simulink model "TENSGwithfourGFM_electromechanical"  (R2020a)
settings: Solver=VariableStepAuto  StartTime=0.0  StopTime=10.0  FixedStep=0.01  RelTol=1e-3
values from neighbouring files (symbols this model uses):
  GFMInit = GFMSimple_init(resultsac,GFM_in_gidx)    [init.m]
  GSGInit =     [SixGFMconfig.mat]    (also in eightGFMconfig.mat; fourGFMconfig.mat; init.m = SG_init(resultsac,SG_in_gidx); tenGFMconfig.mat)
  Pload = [0 0 0 0 0 0 0 0 0 0 0 0 ... (39 elements, 39x1)]    [SixGFMconfig.mat]    (also in eightGFMconfig.mat; fourGFMconfig.mat; init.m = -resultsac.bus{[CZno,CPno],3}/1000; tenGFMconfig.mat)
  Qload = -resultsac.bus{[CZno,CPno],4}/1000    [init.m]
  Satura = Ses_g(GFM_in_gidx)    [init.m]
  U = [1.0278659059 0.919047677638 0.824047236404 0.914672565668 0.984993620745 0.992890253418 1.00337242347 1.00687710353 1.06162588537 0.973548635627 0.980333735458 0.971076509646 ... (88 elements, 88x1)]    [SixGFMconfig.mat]    (also in eightGFMconfig.mat; fourGFMconfig.mat; init.m = resultsac.bus{:,8}.*exp(1i*(resultsac.bus{:,9})/180*pi); tenGFMconfig.mat)
  Vload = Vbus([CZno,CPno])    [init.m]
  W0 = wB    (= 314.159265359)    [init.m]
  Y_new = [-5.55111512313e-17 -2.77555756156e-17 0 0 0 0 0 0 0 0 0 0 ... (7744 elements, 88x88)]    [SixGFMconfig.mat]    (also in eightGFMconfig.mat; fourGFMconfig.mat; init.m = Y_new([CSno,CPno,GFMother],[CSno,CPno,GFMother]); kron.m = Y)
libraries: eeTransforms x53, simulink_extras x10
(part 2 of 3)

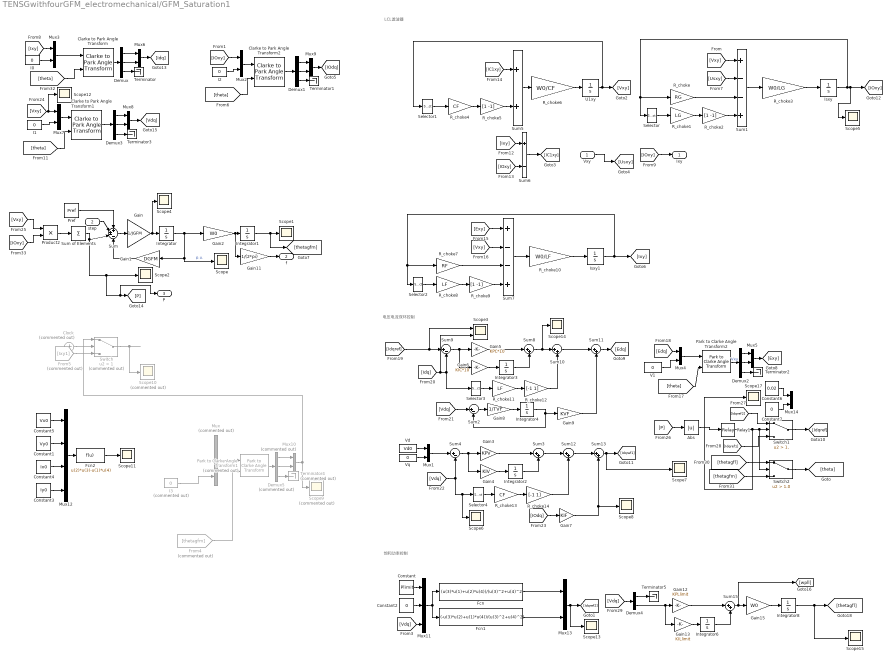
== system TENSGwithfourGFM_electromechanical/GFM_Saturation1 ==
  note: 饱和功率控制
  note: 电压电流双环控制
  note: LCL滤波器
  Vxy : Inport
  step : Inport  Port=2
  Abs : Abs
  Clarke to Park Angle Transform : eeTransforms/Clarke to Park Angle Transform  AxisAlignment=D-axis
      settings: SourceProductBaseCode=PS
  Clarke to Park Angle Transform1 : eeTransforms/Clarke to Park Angle Transform  AxisAlignment=D-axis
      settings: SourceProductBaseCode=PS
  Clarke to Park Angle Transform2 : eeTransforms/Clarke to Park Angle Transform  AxisAlignment=D-axis
      settings: SourceProductBaseCode=PS
  Clock : Clock  Commented=on
  Constant : Constant  Value=Plimit
  Constant1 : Constant  Value=Vy0
  Constant2 : Constant  Value=0
  Constant3 : Constant  Value=Iy0
  Constant4 : Constant  Value=Ix0
  Constant5 : Constant  Value=Vx0
  Constant6 : Constant  Value=0.02
  Constant7 : Constant  Value=0
  Demux{,1..3} (4 alike) : Demux  Outputs=3
  Demux4 : Demux  Outputs=2
  Demux5 : Demux  Commented=on  Outputs=3
  Fcn : Fcn  Expr=(u(3)*u(1)+u(2)*u(4))/(u(3)^2+u(4)^2)
  Fcn1 : Fcn  Expr=(-u(3)*u(2)+u(1)*u(4))/(u(3)^2+u(4)^2)
  Fcn2 : Fcn  Expr=u(2)*u(3)-u(1)*u(4)
  From4 : From  Commented=on  GotoTag=thetagfm
  From5 : From  Commented=on  GotoTag=Ixy1
  Gain : Gain  Gain=1/JGFM
  Gain1 : Gain  Gain=DGFM
  Gain11 : Gain  Gain=1/(2*pi)
  Gain12 : Gain  Gain=KPLlimit
  Gain13 : Gain  Gain=KILlimit
  Gain15 : Gain  Gain=W0
  Gain2 : Gain  Gain=W0
  Gain3 : Gain  Gain=KPV
  Gain4 : Gain  Gain=KIV
  Gain5 : Gain  Gain=KPC*10
  Gain6 : Gain  Gain=KIC*10
  Gain7 : Gain  Gain=KIF
  Gain8 : Gain  Gain=1/TVF
  Gain9 : Gain  Gain=KVF
  I0 : Constant  Value=0
  I1 : Constant  Value=0
  I2 : Constant  Value=0
  I3 : Constant  Commented=on  Value=0
  Integrator : Integrator
  Integrator1 : Integrator  InitialCondition=theta0
  Integrator2 : Integrator  InitialCondition=[Idref0 Iqref0]
  Integrator3 : Integrator  InitialCondition=[Ed0 Eq0]
  Integrator4 : Integrator  InitialCondition=[Vd0 0]
  Integrator6 : Integrator
  Integrator8 : Integrator  InitialCondition=theta0
  Isxy : Integrator  InitialCondition=[IOx0 IOy0]
  Isxy1 : Integrator  InitialCondition=[Ix0 Iy0]
  Mux : Mux  Commented=on  Inputs=3
  Mux{1..9,13..14} (11 alike) : Mux  Inputs=2
  Mux10 : Mux  Commented=on  Inputs=2
  Mux11 : Mux  Inputs=3
  Mux12 : Mux
  Park to Clarke Angle Transform1 : eeTransforms/Park to Clarke Angle Transform  Commented=on  AxisAlignment=D-axis
      settings: SourceProductBaseCode=PS
  Park to Clarke Angle Transform2 : eeTransforms/Park to Clarke Angle Transform  AxisAlignment=D-axis
      settings: SourceProductBaseCode=PS
  Pref : Constant  Value=Pref
  Product2 : Product
  R_choke : Gain  Gain=RG  SaturateOnIntegerOverflow=on  OutDataTypeStr=Inherit: Same as input  ParamDataTypeStr=Inherit: Same as input
  R_choke1 : Gain  Gain=LG  SaturateOnIntegerOverflow=on  OutDataTypeStr=Inherit: Same as input  ParamDataTypeStr=Inherit: Same as input
  R_choke10 : Gain  Gain=W0/LF  SaturateOnIntegerOverflow=on  OutDataTypeStr=Inherit: Same as input  ParamDataTypeStr=Inherit: Same as input
  R_choke11 : Gain  Gain=LF  SaturateOnIntegerOverflow=on  OutDataTypeStr=Inherit: Same as input  ParamDataTypeStr=Inherit: Same as input
  R_choke12 : Gain  Gain=[-1 1]  SaturateOnIntegerOverflow=on  OutDataTypeStr=Inherit: Same as input  ParamDataTypeStr=Inherit: Same as input
  R_choke13 : Gain  Gain=CF  SaturateOnIntegerOverflow=on  OutDataTypeStr=Inherit: Same as input  ParamDataTypeStr=Inherit: Same as input
  R_choke14 : Gain  Gain=[-1 1]  SaturateOnIntegerOverflow=on  OutDataTypeStr=Inherit: Same as input  ParamDataTypeStr=Inherit: Same as input
  R_choke2 : Gain  Gain=[1 -1]  SaturateOnIntegerOverflow=on  OutDataTypeStr=Inherit: Same as input  ParamDataTypeStr=Inherit: Same as input
  R_choke3 : Gain  Gain=W0/LG  SaturateOnIntegerOverflow=on  OutDataTypeStr=Inherit: Same as input  ParamDataTypeStr=Inherit: Same as input
  R_choke4 : Gain  Gain=CF  SaturateOnIntegerOverflow=on  OutDataTypeStr=Inherit: Same as input  ParamDataTypeStr=Inherit: Same as input
  R_choke5 : Gain  Gain=[1 -1]  SaturateOnIntegerOverflow=on  OutDataTypeStr=Inherit: Same as input  ParamDataTypeStr=Inherit: Same as input
  R_choke6 : Gain  Gain=W0/CF  SaturateOnIntegerOverflow=on  OutDataTypeStr=Inherit: Same as input  ParamDataTypeStr=Inherit: Same as input
  R_choke7 : Gain  Gain=RF  SaturateOnIntegerOverflow=on  OutDataTypeStr=Inherit: Same as input  ParamDataTypeStr=Inherit: Same as input
  R_choke8 : Gain  Gain=LF  SaturateOnIntegerOverflow=on  OutDataTypeStr=Inherit: Same as input  ParamDataTypeStr=Inherit: Same as input
  R_choke9 : Gain  Gain=[1 -1]  SaturateOnIntegerOverflow=on  OutDataTypeStr=Inherit: Same as input  ParamDataTypeStr=Inherit: Same as input
  Relay1 : Relay  OnSwitchValue=Plimit  OffSwitchValue=0  OnOutputValue=1.1
  Scope{,1..2,4..8,11..15,17} (14 alike) : Scope
  Scope10 : Scope  Commented=on
  Scope3 : Scope  NumInputPorts=2
  Scope9 : Scope  Commented=on
  Selector{,1..4} (5 alike) : Selector  InputPortWidth=2  IndexOptions=Index vector (dialog)  Indices=[2 1]  OutputSizes=1
  Sum : Sum  Inputs=++--
  Sum of Elements : Sum  Inputs=+
  Sum1 : Sum  Inputs=+--+  SaturateOnIntegerOverflow=on
  Sum{3,8,10..13,15} (7 alike) : Sum  Inputs=|++
  Sum2 : Sum  Inputs=|+-
  Sum4 : Sum  Inputs=|+-
  Sum5 : Sum  SaturateOnIntegerOverflow=on
  Sum6 : Sum  Inputs=+-  SaturateOnIntegerOverflow=on
  Sum7 : Sum  Inputs=+--+  SaturateOnIntegerOverflow=on
  Sum9 : Sum  Inputs=|+-
  Switch : Switch  Commented=on  Criteria=u2 > Threshold  Threshold=1
  Switch1 : Switch  Criteria=u2 > Threshold  Threshold=1.
  Switch2 : Switch  Criteria=u2 > Threshold  Threshold=1.0
  Terminator{,1..3,5} (5 alike) : Terminator
  Terminator4 : Terminator  Commented=on
  U1xy : Integrator  InitialCondition=[Vx0 Vy0]
  V1 : Constant  Value=0
  Vd : Constant  Value=Vd0
  Vq : Constant  Value=0
  Ixy : Outport
  f : Outport  Port=2
  P : Outport  Port=3
  wires:
  Integrator1/1 -> [thetagfm], Scope1/1
  Mux3/1 -> Clarke to Park Angle Transform/1
  I0/1 -> Mux3/2
  Demux/3 -> Terminator/1
  Demux/2 -> Mux6/2
  Gain/1 -> Scope4/1, Integrator/1
  Demux/1 -> Mux6/1
  Clarke to Park Angle Transform/1 -> Demux/1
  Integrator/1 -> Gain2/1, Scope/1, Gain1/1  "p.u."
  Sum of Elements/1 -> Sum/3, P/1, [P], Scope2/1
  Sum/1 -> Gain/1
  Vxy/1 -> [Usxy]
  [Vxy] -> Sum1/1
  [Usxy] -> Sum1/2
  Sum1/1 -> R_choke3/1
  R_choke3/1 -> Isxy/1
  R_choke1/1 -> R_choke2/1
  Isxy/1 -> Scope5/1, [IOxy], R_choke/1, Selector/1
  R_choke/1 -> Sum1/3
  Selector/1 -> R_choke1/1
  R_choke2/1 -> Sum1/4
  [Ixy] -> Mux3/1
  [IOxy] -> Ixy/1
  [theta] -> Clarke to Park Angle Transform/2
  Gain4/1 -> Integrator2/1
  Sum3/1 -> Sum12/1
  Gain3/1 -> Sum3/1
  Integrator2/1 -> Sum3/2
  Sum4/1 -> Gain4/1, Gain3/1
  Vd/1 -> Mux1/1
  Vq/1 -> Mux1/2
  Mux1/1 -> Sum4/1
  R_choke4/1 -> R_choke5/1
  R_choke5/1 -> Sum5/2
  Sum6/1 -> [IC1xy]
  U1xy/1 -> Selector1/1, [Vxy]
  R_choke6/1 -> U1xy/1
  [Ixy] -> Sum6/1
  Selector1/1 -> R_choke4/1
  [IOxy] -> Sum6/2
  [IC1xy] -> Sum5/1
  Sum5/1 -> R_choke6/1
  Isxy1/1 -> [Ixy], R_choke7/1, Selector2/1
  [Vxy] -> Sum7/2
  R_choke7/1 -> Sum7/3
  R_choke8/1 -> R_choke9/1
  R_choke10/1 -> Isxy1/1
  Sum7/1 -> R_choke10/1
  R_choke9/1 -> Sum7/4
  Selector2/1 -> R_choke8/1
  [Edq] -> Mux4/1
  V1/1 -> Mux4/2
  Mux4/1 -> Park to Clarke Angle Transform2/1
  [theta] -> Park to Clarke Angle Transform2/2
  Mux5/1 -> [Exy]
  Demux2/3 -> Terminator2/1
  Park to Clarke Angle Transform2/1 -> Demux2/1  "Vxy"
  Demux2/2 -> Mux5/2
  Demux2/1 -> Mux5/1
  Sum9/1 -> Gain6/1, Gain5/1
  Gain5/1 -> Sum8/1
  Gain6/1 -> Integrator3/1
  Integrator3/1 -> Sum8/2
  R_choke11/1 -> R_choke12/1
  Selector3/1 -> R_choke11/1
  Sum8/1 -> Scope14/1, Sum10/1
  R_choke12/1 -> Sum10/2
  Sum10/1 -> Sum11/1
  Gain9/1 -> Sum11/2
  Sum11/1 -> [Edq]
  Selector4/1 -> R_choke13/1
  [Vdq] -> Scope6/1, Selector4/1, Sum4/2
  R_choke13/1 -> R_choke14/1
  R_choke14/1 -> Sum12/2
  Sum12/1 -> Sum13/1
  Sum13/1 -> Scope7/1, [Idqref1]
  [IOdq] -> Gain7/1
  Gain7/1 -> Sum13/2, Scope8/1
  Mux6/1 -> [Idq]
  [Vxy] -> Scope12/1, Mux7/1
  I1/1 -> Mux7/2
  Mux7/1 -> Clarke to Park Angle Transform1/1
  [theta] -> Clarke to Park Angle Transform1/2
  Clarke to Park Angle Transform1/1 -> Demux3/1
  Demux3/1 -> Mux8/1
  Demux3/2 -> Mux8/2
  Mux8/1 -> [Vdq]
  Demux3/3 -> Terminator3/1
  [theta] -> Clarke to Park Angle Transform2/2
  Clarke to Park Angle Transform2/1 -> Demux1/1
  Demux1/1 -> Mux9/1
  Demux1/2 -> Mux9/2
  [IOxy] -> Mux2/1
  Demux1/3 -> Terminator1/1
  Mux2/1 -> Clarke to Park Angle Transform2/1
  Mux9/1 -> [IOdq]
  I2/1 -> Mux2/2
  [Vxy] -> Product2/1
  [IOxy] -> Product2/2
  Product2/1 -> Sum of Elements/1
  Sum2/1 -> Gain8/1
  Integrator4/1 -> Gain9/1, Sum2/2
  Gain8/1 -> Integrator4/1
  [Vdq] -> Sum2/1
  [Exy] -> Sum7/1
  Gain2/1 -> Gain11/1, Integrator1/1
  Gain11/1 -> f/1
  Pref/1 -> Sum/1
  [Idq] -> Sum9/2, Selector3/1, Scope3/2
  Demux5/3 -> Terminator4/1
  Mux/1 -> Park to Clarke Angle Transform1/1
  Demux5/2 -> Mux10/2
  Park to Clarke Angle Transform1/1 -> Demux5/1
  Mux10/1 -> Scope9/1, Switch/1
  Demux5/1 -> Mux10/1
  I3/1 -> Mux/3
  [Idqref] -> Scope3/1, Sum9/1
  Switch/1 -> Scope10/1
  From5/1 -> Switch/3
  Clock/1 -> Switch/2
  From4/1 -> Park to Clarke Angle Transform1/2
  Mux11/1 -> Fcn1/1, Fcn/1
  Constant/1 -> Mux11/1
  Constant5/1 -> Mux12/1
  Constant1/1 -> Mux12/2
  Constant4/1 -> Mux12/3
  Constant3/1 -> Mux12/4
  Mux12/1 -> Fcn2/1
  Constant2/1 -> Mux11/2
  Fcn2/1 -> Scope11/1
  Mux13/1 -> Scope13/1, [Idqref2]
  [P] -> Abs/1
  Relay1/1 -> Scope17/1, Switch1/2, Switch2/2
  Switch1/1 -> [Idqref]
  [Idqref1] -> Switch1/3
  Integrator6/1 -> Sum15/2
  Gain13/1 -> Integrator6/1
  Demux4/1 -> Terminator5/1
  Gain15/1 -> Integrator8/1
  [Vdq] -> Demux4/1
  Demux4/2 -> Gain13/1, Gain12/1
  Integrator8/1 -> Scope15/1, [thetagfl]
  Gain12/1 -> Sum15/1
  [thetagfl] -> Switch2/1
  [thetagfm] -> Switch2/3
  Switch2/1 -> [theta]
  Fcn/1 -> Mux13/1
  Fcn1/1 -> Mux13/2
  [Vdq] -> Mux11/3
  Constant6/1 -> Mux14/1
  Constant7/1 -> Mux14/2
  [Idqref2] -> Switch1/1
  Sum15/1 -> [wpll], Gain15/1
  Abs/1 -> Relay1/1
  Gain1/1 -> Sum/4
  step/1 -> Sum/2

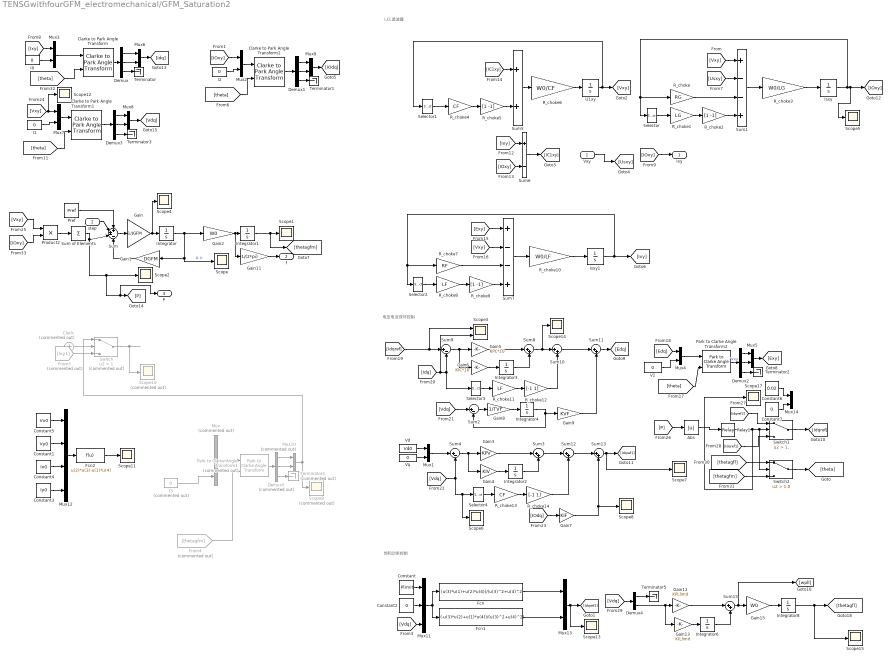
== system TENSGwithfourGFM_electromechanical/GFM_Saturation2 ==
  note: LCL滤波器
  note: 电压电流双环控制
  note: 饱和功率控制
  Vxy : Inport
  step : Inport  Port=2
  Abs : Abs
  Clarke to Park Angle Transform : eeTransforms/Clarke to Park Angle Transform  AxisAlignment=D-axis
      settings: SourceProductBaseCode=PS
  Clarke to Park Angle Transform1 : eeTransforms/Clarke to Park Angle Transform  AxisAlignment=D-axis
      settings: SourceProductBaseCode=PS
  Clarke to Park Angle Transform2 : eeTransforms/Clarke to Park Angle Transform  AxisAlignment=D-axis
      settings: SourceProductBaseCode=PS
  Clock : Clock  Commented=on
  Constant : Constant  Value=Plimit
  Constant1 : Constant  Value=Vy0
  Constant2 : Constant  Value=0
  Constant3 : Constant  Value=Iy0
  Constant4 : Constant  Value=Ix0
  Constant5 : Constant  Value=Vx0
  Constant6 : Constant  Value=0.02
  Constant7 : Constant  Value=0
  Demux{,1..3} (4 alike) : Demux  Outputs=3
  Demux4 : Demux  Outputs=2
  Demux5 : Demux  Commented=on  Outputs=3
  Fcn : Fcn  Expr=(u(3)*u(1)+u(2)*u(4))/(u(3)^2+u(4)^2)
  Fcn1 : Fcn  Expr=(-u(3)*u(2)+u(1)*u(4))/(u(3)^2+u(4)^2)
  Fcn2 : Fcn  Expr=u(2)*u(3)-u(1)*u(4)
  From4 : From  Commented=on  GotoTag=thetagfm
  From5 : From  Commented=on  GotoTag=Ixy1
  Gain : Gain  Gain=1/JGFM
  Gain1 : Gain  Gain=DGFM
  Gain11 : Gain  Gain=1/(2*pi)
  Gain12 : Gain  Gain=KPLlimit
  Gain13 : Gain  Gain=KILlimit
  Gain15 : Gain  Gain=W0
  Gain2 : Gain  Gain=W0
  Gain3 : Gain  Gain=KPV
  Gain4 : Gain  Gain=KIV
  Gain5 : Gain  Gain=KPC*10
  Gain6 : Gain  Gain=KIC*10
  Gain7 : Gain  Gain=KIF
  Gain8 : Gain  Gain=1/TVF
  Gain9 : Gain  Gain=KVF
  I0 : Constant  Value=0
  I1 : Constant  Value=0
  I2 : Constant  Value=0
  I3 : Constant  Commented=on  Value=0
  Integrator : Integrator
  Integrator1 : Integrator  InitialCondition=theta0
  Integrator2 : Integrator  InitialCondition=[Idref0 Iqref0]
  Integrator3 : Integrator  InitialCondition=[Ed0 Eq0]
  Integrator4 : Integrator  InitialCondition=[Vd0 0]
  Integrator6 : Integrator
  Integrator8 : Integrator  InitialCondition=theta0
  Isxy : Integrator  InitialCondition=[IOx0 IOy0]
  Isxy1 : Integrator  InitialCondition=[Ix0 Iy0]
  Mux : Mux  Commented=on  Inputs=3
  Mux{1..9,13..14} (11 alike) : Mux  Inputs=2
  Mux10 : Mux  Commented=on  Inputs=2
  Mux11 : Mux  Inputs=3
  Mux12 : Mux
  Park to Clarke Angle Transform1 : eeTransforms/Park to Clarke Angle Transform  Commented=on  AxisAlignment=D-axis
      settings: SourceProductBaseCode=PS
  Park to Clarke Angle Transform2 : eeTransforms/Park to Clarke Angle Transform  AxisAlignment=D-axis
      settings: SourceProductBaseCode=PS
  Pref : Constant  Value=Pref
  Product2 : Product
  R_choke : Gain  Gain=RG  SaturateOnIntegerOverflow=on  OutDataTypeStr=Inherit: Same as input  ParamDataTypeStr=Inherit: Same as input
  R_choke1 : Gain  Gain=LG  SaturateOnIntegerOverflow=on  OutDataTypeStr=Inherit: Same as input  ParamDataTypeStr=Inherit: Same as input
  R_choke10 : Gain  Gain=W0/LF  SaturateOnIntegerOverflow=on  OutDataTypeStr=Inherit: Same as input  ParamDataTypeStr=Inherit: Same as input
  R_choke11 : Gain  Gain=LF  SaturateOnIntegerOverflow=on  OutDataTypeStr=Inherit: Same as input  ParamDataTypeStr=Inherit: Same as input
  R_choke12 : Gain  Gain=[-1 1]  SaturateOnIntegerOverflow=on  OutDataTypeStr=Inherit: Same as input  ParamDataTypeStr=Inherit: Same as input
  R_choke13 : Gain  Gain=CF  SaturateOnIntegerOverflow=on  OutDataTypeStr=Inherit: Same as input  ParamDataTypeStr=Inherit: Same as input
  R_choke14 : Gain  Gain=[-1 1]  SaturateOnIntegerOverflow=on  OutDataTypeStr=Inherit: Same as input  ParamDataTypeStr=Inherit: Same as input
  R_choke2 : Gain  Gain=[1 -1]  SaturateOnIntegerOverflow=on  OutDataTypeStr=Inherit: Same as input  ParamDataTypeStr=Inherit: Same as input
  R_choke3 : Gain  Gain=W0/LG  SaturateOnIntegerOverflow=on  OutDataTypeStr=Inherit: Same as input  ParamDataTypeStr=Inherit: Same as input
  R_choke4 : Gain  Gain=CF  SaturateOnIntegerOverflow=on  OutDataTypeStr=Inherit: Same as input  ParamDataTypeStr=Inherit: Same as input
  R_choke5 : Gain  Gain=[1 -1]  SaturateOnIntegerOverflow=on  OutDataTypeStr=Inherit: Same as input  ParamDataTypeStr=Inherit: Same as input
  R_choke6 : Gain  Gain=W0/CF  SaturateOnIntegerOverflow=on  OutDataTypeStr=Inherit: Same as input  ParamDataTypeStr=Inherit: Same as input
  R_choke7 : Gain  Gain=RF  SaturateOnIntegerOverflow=on  OutDataTypeStr=Inherit: Same as input  ParamDataTypeStr=Inherit: Same as input
  R_choke8 : Gain  Gain=LF  SaturateOnIntegerOverflow=on  OutDataTypeStr=Inherit: Same as input  ParamDataTypeStr=Inherit: Same as input
  R_choke9 : Gain  Gain=[1 -1]  SaturateOnIntegerOverflow=on  OutDataTypeStr=Inherit: Same as input  ParamDataTypeStr=Inherit: Same as input
  Relay1 : Relay  OnSwitchValue=Plimit  OffSwitchValue=0  OnOutputValue=1.1
  Scope{,1..2,4..8,11..15,17} (14 alike) : Scope
  Scope10 : Scope  Commented=on
  Scope3 : Scope  NumInputPorts=2
  Scope9 : Scope  Commented=on
  Selector{,1..4} (5 alike) : Selector  InputPortWidth=2  IndexOptions=Index vector (dialog)  Indices=[2 1]  OutputSizes=1
  Sum : Sum  Inputs=++--
  Sum of Elements : Sum  Inputs=+
  Sum1 : Sum  Inputs=+--+  SaturateOnIntegerOverflow=on
  Sum{3,8,10..13,15} (7 alike) : Sum  Inputs=|++
  Sum2 : Sum  Inputs=|+-
  Sum4 : Sum  Inputs=|+-
  Sum5 : Sum  SaturateOnIntegerOverflow=on
  Sum6 : Sum  Inputs=+-  SaturateOnIntegerOverflow=on
  Sum7 : Sum  Inputs=+--+  SaturateOnIntegerOverflow=on
  Sum9 : Sum  Inputs=|+-
  Switch : Switch  Commented=on  Criteria=u2 > Threshold  Threshold=1
  Switch1 : Switch  Criteria=u2 > Threshold  Threshold=1.
  Switch2 : Switch  Criteria=u2 > Threshold  Threshold=1.0
  Terminator{,1..3,5} (5 alike) : Terminator
  Terminator4 : Terminator  Commented=on
  U1xy : Integrator  InitialCondition=[Vx0 Vy0]
  V1 : Constant  Value=0
  Vd : Constant  Value=Vd0
  Vq : Constant  Value=0
  Ixy : Outport
  f : Outport  Port=2
  P : Outport  Port=3
  wires:
  step/1 -> Sum/2
  Gain1/1 -> Sum/4
  Abs/1 -> Relay1/1
  Sum15/1 -> Gain15/1, [wpll]
  [Idqref2] -> Switch1/1
  Constant7/1 -> Mux14/2
  Constant6/1 -> Mux14/1
  [Vdq] -> Mux11/3
  Fcn1/1 -> Mux13/2
  Fcn/1 -> Mux13/1
  Switch2/1 -> [theta]
  [thetagfm] -> Switch2/3
  [thetagfl] -> Switch2/1
  Gain12/1 -> Sum15/1
  Integrator8/1 -> [thetagfl], Scope15/1
  Demux4/2 -> Gain12/1, Gain13/1
  [Vdq] -> Demux4/1
  Gain15/1 -> Integrator8/1
  Demux4/1 -> Terminator5/1
  Gain13/1 -> Integrator6/1
  Integrator6/1 -> Sum15/2
  [Idqref1] -> Switch1/3
  Switch1/1 -> [Idqref]
  Relay1/1 -> Switch2/2, Switch1/2, Scope17/1
  [P] -> Abs/1
  Mux13/1 -> [Idqref2], Scope13/1
  Fcn2/1 -> Scope11/1
  Constant2/1 -> Mux11/2
  Mux12/1 -> Fcn2/1
  Constant3/1 -> Mux12/4
  Constant4/1 -> Mux12/3
  Constant1/1 -> Mux12/2
  Constant5/1 -> Mux12/1
  Constant/1 -> Mux11/1
  Mux11/1 -> Fcn/1, Fcn1/1
  From4/1 -> Park to Clarke Angle Transform1/2
  Clock/1 -> Switch/2
  From5/1 -> Switch/3
  Switch/1 -> Scope10/1
  [Idqref] -> Sum9/1, Scope3/1
  I3/1 -> Mux/3
  Demux5/1 -> Mux10/1
  Mux10/1 -> Switch/1, Scope9/1
  Park to Clarke Angle Transform1/1 -> Demux5/1
  Demux5/2 -> Mux10/2
  Mux/1 -> Park to Clarke Angle Transform1/1
  Demux5/3 -> Terminator4/1
  [Idq] -> Scope3/2, Selector3/1, Sum9/2
  Pref/1 -> Sum/1
  Gain11/1 -> f/1
  Gain2/1 -> Integrator1/1, Gain11/1
  [Exy] -> Sum7/1
  [Vdq] -> Sum2/1
  Gain8/1 -> Integrator4/1
  Integrator4/1 -> Sum2/2, Gain9/1
  Sum2/1 -> Gain8/1
  Product2/1 -> Sum of Elements/1
  [IOxy] -> Product2/2
  [Vxy] -> Product2/1
  I2/1 -> Mux2/2
  Mux9/1 -> [IOdq]
  Mux2/1 -> Clarke to Park Angle Transform2/1
  Demux1/3 -> Terminator1/1
  [IOxy] -> Mux2/1
  Demux1/2 -> Mux9/2
  Demux1/1 -> Mux9/1
  Clarke to Park Angle Transform2/1 -> Demux1/1
  [theta] -> Clarke to Park Angle Transform2/2
  Demux3/3 -> Terminator3/1
  Mux8/1 -> [Vdq]
  Demux3/2 -> Mux8/2
  Demux3/1 -> Mux8/1
  Clarke to Park Angle Transform1/1 -> Demux3/1
  [theta] -> Clarke to Park Angle Transform1/2
  Mux7/1 -> Clarke to Park Angle Transform1/1
  I1/1 -> Mux7/2
  [Vxy] -> Mux7/1, Scope12/1
  Mux6/1 -> [Idq]
  Gain7/1 -> Scope8/1, Sum13/2
  [IOdq] -> Gain7/1
  Sum13/1 -> [Idqref1], Scope7/1
  Sum12/1 -> Sum13/1
  R_choke14/1 -> Sum12/2
  R_choke13/1 -> R_choke14/1
  [Vdq] -> Sum4/2, Selector4/1, Scope6/1
  Selector4/1 -> R_choke13/1
  Sum11/1 -> [Edq]
  Gain9/1 -> Sum11/2
  Sum10/1 -> Sum11/1
  R_choke12/1 -> Sum10/2
  Sum8/1 -> Sum10/1, Scope14/1
  Selector3/1 -> R_choke11/1
  R_choke11/1 -> R_choke12/1
  Integrator3/1 -> Sum8/2
  Gain6/1 -> Integrator3/1
  Gain5/1 -> Sum8/1
  Sum9/1 -> Gain5/1, Gain6/1
  Demux2/1 -> Mux5/1
  Demux2/2 -> Mux5/2
  Park to Clarke Angle Transform2/1 -> Demux2/1  "Vxy"
  Demux2/3 -> Terminator2/1
  Mux5/1 -> [Exy]
  [theta] -> Park to Clarke Angle Transform2/2
  Mux4/1 -> Park to Clarke Angle Transform2/1
  V1/1 -> Mux4/2
  [Edq] -> Mux4/1
  Selector2/1 -> R_choke8/1
  R_choke9/1 -> Sum7/4
  Sum7/1 -> R_choke10/1
  R_choke10/1 -> Isxy1/1
  R_choke8/1 -> R_choke9/1
  R_choke7/1 -> Sum7/3
  [Vxy] -> Sum7/2
  Isxy1/1 -> Selector2/1, R_choke7/1, [Ixy]
  Sum5/1 -> R_choke6/1
  [IC1xy] -> Sum5/1
  [IOxy] -> Sum6/2
  Selector1/1 -> R_choke4/1
  [Ixy] -> Sum6/1
  R_choke6/1 -> U1xy/1
  U1xy/1 -> [Vxy], Selector1/1
  Sum6/1 -> [IC1xy]
  R_choke5/1 -> Sum5/2
  R_choke4/1 -> R_choke5/1
  Mux1/1 -> Sum4/1
  Vq/1 -> Mux1/2
  Vd/1 -> Mux1/1
  Sum4/1 -> Gain3/1, Gain4/1
  Integrator2/1 -> Sum3/2
  Gain3/1 -> Sum3/1
  Sum3/1 -> Sum12/1
  Gain4/1 -> Integrator2/1
  [theta] -> Clarke to Park Angle Transform/2
  [IOxy] -> Ixy/1
  [Ixy] -> Mux3/1
  R_choke2/1 -> Sum1/4
  Selector/1 -> R_choke1/1
  R_choke/1 -> Sum1/3
  Isxy/1 -> Selector/1, R_choke/1, [IOxy], Scope5/1
  R_choke1/1 -> R_choke2/1
  R_choke3/1 -> Isxy/1
  Sum1/1 -> R_choke3/1
  [Usxy] -> Sum1/2
  [Vxy] -> Sum1/1
  Vxy/1 -> [Usxy]
  Sum/1 -> Gain/1
  Sum of Elements/1 -> Scope2/1, [P], P/1, Sum/3
  Integrator/1 -> Gain1/1, Scope/1, Gain2/1  "p.u."
  Clarke to Park Angle Transform/1 -> Demux/1
  Demux/1 -> Mux6/1
  Gain/1 -> Integrator/1, Scope4/1
  Demux/2 -> Mux6/2
  Demux/3 -> Terminator/1
  I0/1 -> Mux3/2
  Mux3/1 -> Clarke to Park Angle Transform/1
  Integrator1/1 -> Scope1/1, [thetagfm]

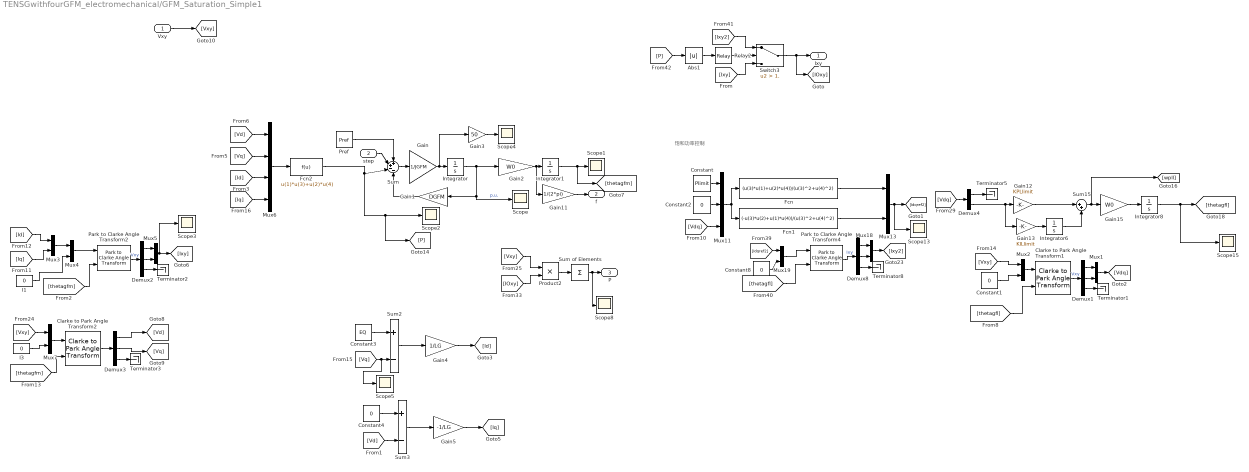
== system TENSGwithfourGFM_electromechanical/GFM_Saturation_Simple1 ==
  note: 饱和功率控制
  Vxy : Inport
  step : Inport  Port=2
  Abs1 : Abs
  Clarke to Park Angle Transform1 : eeTransforms/Clarke to Park Angle Transform  AxisAlignment=D-axis
      settings: SourceProductBaseCode=PS
  Clarke to Park Angle Transform2 : eeTransforms/Clarke to Park Angle Transform  AxisAlignment=D-axis
      settings: SourceProductBaseCode=PS
  Constant : Constant  Value=Plimit
  Constant{1..2,4,8} (4 alike) : Constant  Value=0
  Constant3 : Constant  Value=EQ
  Demux{1..3,8} (4 alike) : Demux  Outputs=3
  Demux4 : Demux  Outputs=2
  Fcn : Fcn  Expr=(u(3)*u(1)+u(2)*u(4))/(u(3)^2+u(4)^2)
  Fcn1 : Fcn  Expr=(-u(3)*u(2)+u(1)*u(4))/(u(3)^2+u(4)^2)
  Fcn2 : Fcn  Expr=u(1)*u(3)+u(2)*u(4)
  Gain : Gain  Gain=1/JGFM
  Gain1 : Gain  Gain=DGFM
  Gain11 : Gain  Gain=1/(2*pi)
  Gain12 : Gain  Gain=KPLlimit
  Gain13 : Gain  Gain=KILlimit
  Gain15 : Gain  Gain=W0
  Gain2 : Gain  Gain=W0
  Gain3 : Gain  Gain=50
  Gain4 : Gain  Gain=1/LG
  Gain5 : Gain  Gain=-1/LG
  I1 : Constant  Value=0
  I3 : Constant  Value=0
  Integrator : Integrator
  Integrator1 : Integrator  InitialCondition=theta0
  Integrator6 : Integrator
  Integrator8 : Integrator  InitialCondition=theta0
  Mux{1..5,7,13,18..19} (9 alike) : Mux  Inputs=2
  Mux11 : Mux  Inputs=3
  Mux6 : Mux
  Park to Clarke Angle Transform2 : eeTransforms/Park to Clarke Angle Transform  AxisAlignment=D-axis
      settings: SourceProductBaseCode=PS
  Park to Clarke Angle Transform4 : eeTransforms/Park to Clarke Angle Transform  AxisAlignment=D-axis
      settings: SourceProductBaseCode=PS
  Pref : Constant  Value=Pref
  Product2 : Product
  Relay2 : Relay  OnSwitchValue=Plimit  OffSwitchValue=0  OnOutputValue=1.1
  Scope{,1..5,8,13,15} (9 alike) : Scope
  Sum : Sum  Inputs=++--
  Sum of Elements : Sum  Inputs=+
  Sum15 : Sum  Inputs=|++
  Sum2 : Sum  Inputs=+-  SaturateOnIntegerOverflow=on
  Sum3 : Sum  Inputs=+-  SaturateOnIntegerOverflow=on
  Switch3 : Switch  Criteria=u2 > Threshold  Threshold=1.
  Terminator{1..3,5,8} (5 alike) : Terminator
  Ixy : Outport
  f : Outport  Port=2
  P : Outport  Port=3
  wires:
  Integrator1/1 -> [thetagfm], Scope1/1
  Gain/1 -> Gain3/1, Integrator/1
  Integrator/1 -> Gain2/1, Scope/1, Gain1/1  "p.u."
  Fcn2/1 -> Sum/3, [P], Scope2/1
  Sum/1 -> Gain/1
  Vxy/1 -> [Vxy]
  Gain2/1 -> Gain11/1, Integrator1/1
  Gain11/1 -> f/1
  Pref/1 -> Sum/1
  Mux11/1 -> Fcn1/1, Fcn/1
  Constant/1 -> Mux11/1
  Constant2/1 -> Mux11/2
  Mux13/1 -> Scope13/1, [Idqref2]
  Integrator6/1 -> Sum15/2
  Gain13/1 -> Integrator6/1
  Demux4/1 -> Terminator5/1
  Gain15/1 -> Integrator8/1
  [Vdq] -> Demux4/1
  Demux4/2 -> Gain13/1, Gain12/1
  Integrator8/1 -> Scope15/1, [thetagfl]
  Gain12/1 -> Sum15/1
  Fcn/1 -> Mux13/1
  Fcn1/1 -> Mux13/2
  [Vdq] -> Mux11/3
  Sum15/1 -> [wpll], Gain15/1
  Gain1/1 -> Sum/4
  step/1 -> Sum/2
  Demux8/3 -> Terminator8/1
  Mux18/1 -> [Ixy2]
  Park to Clarke Angle Transform4/1 -> Demux8/1  "Ixy"
  Demux8/2 -> Mux18/2
  Demux8/1 -> Mux18/1
  [Idqref2] -> Mux19/1
  Constant8/1 -> Mux19/2
  Mux19/1 -> Park to Clarke Angle Transform4/1
  [thetagfl] -> Park to Clarke Angle Transform4/2
  [P] -> Abs1/1
  Abs1/1 -> Relay2/1
  Relay2/1 -> Switch3/2
  [Ixy2] -> Switch3/1
  [Ixy] -> Switch3/3
  Switch3/1 -> [IOxy], Ixy/1
  [Vxy] -> Mux2/1
  Constant1/1 -> Mux2/2
  Mux2/1 -> Clarke to Park Angle Transform1/1
  [thetagfl] -> Clarke to Park Angle Transform1/2
  Demux1/3 -> Terminator1/1
  Mux1/1 -> [Vdq]
  Clarke to Park Angle Transform1/1 -> Demux1/1  "Vxy"
  Demux1/2 -> Mux1/2
  Demux1/1 -> Mux1/1
  Gain3/1 -> Scope4/1
  Constant3/1 -> Sum2/1
  [Vq] -> Scope5/1, Sum2/2
  Sum2/1 -> Gain4/1
  Gain4/1 -> [Id]
  Sum3/1 -> Gain5/1
  Constant4/1 -> Sum3/1
  [Vd] -> Sum3/2
  Gain5/1 -> [Iq]
  Demux2/3 -> Terminator2/1
  Demux3/1 -> [Vd]
  [thetagfm] -> Clarke to Park Angle Transform2/2
  Park to Clarke Angle Transform2/1 -> Demux2/1  "Vxy"
  Demux2/2 -> Mux5/2
  Mux4/1 -> Park to Clarke Angle Transform2/1
  Demux3/2 -> [Vq]
  Demux3/3 -> Terminator3/1
  I3/1 -> Mux7/2
  Demux2/1 -> Mux5/1
  Clarke to Park Angle Transform2/1 -> Demux3/1
  Mux5/1 -> [Ixy], Scope3/1
  [thetagfm] -> Park to Clarke Angle Transform2/2
  [Vxy] -> Mux7/1
  Mux7/1 -> Clarke to Park Angle Transform2/1
  [Id] -> Mux3/1
  [Iq] -> Mux3/2
  Mux3/1 -> Mux4/1
  I1/1 -> Mux4/2
  [Id] -> Mux6/3
  [Vd] -> Mux6/1
  Mux6/1 -> Fcn2/1
  [Vq] -> Mux6/2
  [Iq] -> Mux6/4
  [IOxy] -> Product2/2
  Product2/1 -> Sum of Elements/1
  Sum of Elements/1 -> Scope8/1, P/1
  [Vxy] -> Product2/1

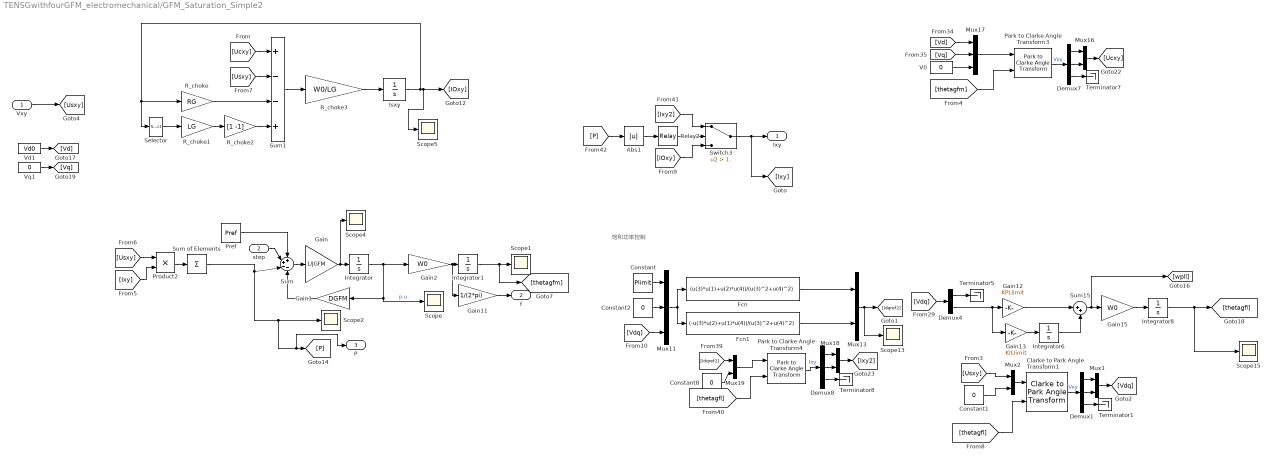
== system TENSGwithfourGFM_electromechanical/GFM_Saturation_Simple2 ==
  note: 饱和功率控制
  Vxy : Inport
  step : Inport  Port=2
  Abs1 : Abs
  Clarke to Park Angle Transform1 : eeTransforms/Clarke to Park Angle Transform  AxisAlignment=D-axis
      settings: SourceProductBaseCode=PS
  Constant : Constant  Value=Plimit
  Constant1 : Constant  Value=0
  Constant2 : Constant  Value=0
  Constant8 : Constant  Value=0
  Demux1 : Demux  Outputs=3
  Demux4 : Demux  Outputs=2
  Demux7 : Demux  Outputs=3
  Demux8 : Demux  Outputs=3
  Fcn : Fcn  Expr=(u(3)*u(1)+u(2)*u(4))/(u(3)^2+u(4)^2)
  Fcn1 : Fcn  Expr=(-u(3)*u(2)+u(1)*u(4))/(u(3)^2+u(4)^2)
  Gain : Gain  Gain=1/JGFM
  Gain1 : Gain  Gain=DGFM
  Gain11 : Gain  Gain=1/(2*pi)
  Gain12 : Gain  Gain=KPLlimit
  Gain13 : Gain  Gain=KILlimit
  Gain15 : Gain  Gain=W0
  Gain2 : Gain  Gain=W0
  Integrator : Integrator
  Integrator1 : Integrator  InitialCondition=theta0
  Integrator6 : Integrator
  Integrator8 : Integrator  InitialCondition=theta0
  Isxy : Integrator  InitialCondition=[IOx0 IOy0]
  Mux{1..2,13,16,18..19} (6 alike) : Mux  Inputs=2
  Mux11 : Mux  Inputs=3
  Mux17 : Mux  Inputs=3
  Park to Clarke Angle Transform3 : eeTransforms/Park to Clarke Angle Transform  AxisAlignment=D-axis
      settings: SourceProductBaseCode=PS
  Park to Clarke Angle Transform4 : eeTransforms/Park to Clarke Angle Transform  AxisAlignment=D-axis
      settings: SourceProductBaseCode=PS
  Pref : Constant  Value=Pref
  Product2 : Product
  R_choke : Gain  Gain=RG  SaturateOnIntegerOverflow=on  OutDataTypeStr=Inherit: Same as input  ParamDataTypeStr=Inherit: Same as input
  R_choke1 : Gain  Gain=LG  SaturateOnIntegerOverflow=on  OutDataTypeStr=Inherit: Same as input  ParamDataTypeStr=Inherit: Same as input
  R_choke2 : Gain  Gain=[1 -1]  SaturateOnIntegerOverflow=on  OutDataTypeStr=Inherit: Same as input  ParamDataTypeStr=Inherit: Same as input
  R_choke3 : Gain  Gain=W0/LG  SaturateOnIntegerOverflow=on  OutDataTypeStr=Inherit: Same as input  ParamDataTypeStr=Inherit: Same as input
  Relay2 : Relay  OnSwitchValue=Plimit  OffSwitchValue=0  OnOutputValue=1.1
  Scope{,1..2,4..5,13,15} (7 alike) : Scope
  Selector : Selector  InputPortWidth=2  IndexOptions=Index vector (dialog)  Indices=[2 1]  OutputSizes=1
  Sum : Sum  Inputs=++--
  Sum of Elements : Sum  Inputs=+
  Sum1 : Sum  Inputs=+--+  SaturateOnIntegerOverflow=on
  Sum15 : Sum  Inputs=|++
  Switch3 : Switch  Criteria=u2 > Threshold  Threshold=1.
  Terminator{1,5,7..8} (4 alike) : Terminator
  V0 : Constant  Value=0
  Vd1 : Constant  Value=Vd0
  Vq1 : Constant  Value=0
  Ixy : Outport
  f : Outport  Port=2
  P : Outport  Port=3
  wires:
  Integrator1/1 -> [thetagfm], Scope1/1
  Gain/1 -> Scope4/1, Integrator/1
  Integrator/1 -> Gain2/1, Scope/1, Gain1/1  "p.u."
  Sum of Elements/1 -> Sum/3, P/1, [P], Scope2/1
  Sum/1 -> Gain/1
  Vxy/1 -> [Usxy]
  [Ucxy] -> Sum1/1
  [Usxy] -> Sum1/2
  Sum1/1 -> R_choke3/1
  R_choke3/1 -> Isxy/1
  R_choke1/1 -> R_choke2/1
  Isxy/1 -> Scope5/1, [IOxy], R_choke/1, Selector/1
  R_choke/1 -> Sum1/3
  Selector/1 -> R_choke1/1
  R_choke2/1 -> Sum1/4
  Gain2/1 -> Gain11/1, Integrator1/1
  Gain11/1 -> f/1
  Pref/1 -> Sum/1
  Mux11/1 -> Fcn1/1, Fcn/1
  Constant/1 -> Mux11/1
  Constant2/1 -> Mux11/2
  Mux13/1 -> Scope13/1, [Idqref2]
  Integrator6/1 -> Sum15/2
  Gain13/1 -> Integrator6/1
  Demux4/1 -> Terminator5/1
  Gain15/1 -> Integrator8/1
  [Vdq] -> Demux4/1
  Demux4/2 -> Gain13/1, Gain12/1
  Integrator8/1 -> Scope15/1, [thetagfl]
  Gain12/1 -> Sum15/1
  Fcn/1 -> Mux13/1
  Fcn1/1 -> Mux13/2
  [Vdq] -> Mux11/3
  Sum15/1 -> [wpll], Gain15/1
  Gain1/1 -> Sum/4
  step/1 -> Sum/2
  Vq1/1 -> [Vq]
  Vd1/1 -> [Vd]
  Demux7/1 -> Mux16/1
  [Vq] -> Mux17/2
  Demux7/2 -> Mux16/2
  Mux16/1 -> [Ucxy]
  Park to Clarke Angle Transform3/1 -> Demux7/1  "Vxy"
  Mux17/1 -> Park to Clarke Angle Transform3/1
  V0/1 -> Mux17/3
  [Vd] -> Mux17/1
  Demux7/3 -> Terminator7/1
  [thetagfm] -> Park to Clarke Angle Transform3/2
  Demux8/3 -> Terminator8/1
  Mux18/1 -> [Ixy2]
  Park to Clarke Angle Transform4/1 -> Demux8/1  "Ixy"
  Demux8/2 -> Mux18/2
  Demux8/1 -> Mux18/1
  [Idqref2] -> Mux19/1
  Constant8/1 -> Mux19/2
  Mux19/1 -> Park to Clarke Angle Transform4/1
  [thetagfl] -> Park to Clarke Angle Transform4/2
  [P] -> Abs1/1
  Abs1/1 -> Relay2/1
  Relay2/1 -> Switch3/2
  [Ixy2] -> Switch3/1
  [IOxy] -> Switch3/3
  Switch3/1 -> [Ixy], Ixy/1
  [Usxy] -> Product2/1
  [Ixy] -> Product2/2
  Product2/1 -> Sum of Elements/1
  [Usxy] -> Mux2/1
  Constant1/1 -> Mux2/2
  Mux2/1 -> Clarke to Park Angle Transform1/1
  [thetagfl] -> Clarke to Park Angle Transform1/2
  Demux1/3 -> Terminator1/1
  Mux1/1 -> [Vdq]
  Clarke to Park Angle Transform1/1 -> Demux1/1  "Vxy"
  Demux1/2 -> Mux1/2
  Demux1/1 -> Mux1/1

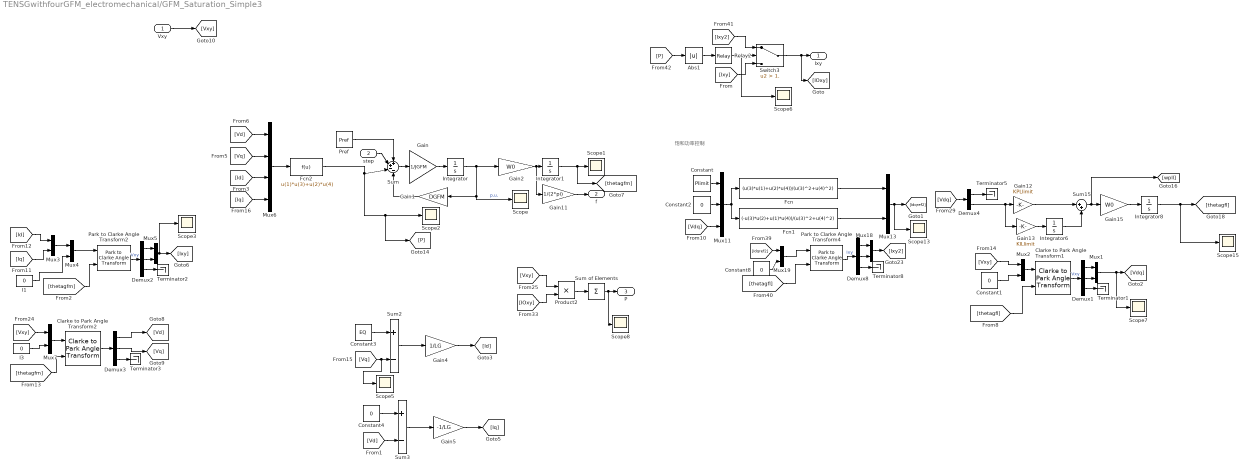
== system TENSGwithfourGFM_electromechanical/GFM_Saturation_Simple3 ==
  note: 饱和功率控制
  Vxy : Inport
  step : Inport  Port=2
  Abs1 : Abs
  Clarke to Park Angle Transform1 : eeTransforms/Clarke to Park Angle Transform  AxisAlignment=D-axis
      settings: SourceProductBaseCode=PS
  Clarke to Park Angle Transform2 : eeTransforms/Clarke to Park Angle Transform  AxisAlignment=D-axis
      settings: SourceProductBaseCode=PS
  Constant : Constant  Value=Plimit
  Constant{1..2,4,8} (4 alike) : Constant  Value=0
  Constant3 : Constant  Value=EQ
  Demux{1..3,8} (4 alike) : Demux  Outputs=3
  Demux4 : Demux  Outputs=2
  Fcn : Fcn  Expr=(u(3)*u(1)+u(2)*u(4))/(u(3)^2+u(4)^2)
  Fcn1 : Fcn  Expr=(-u(3)*u(2)+u(1)*u(4))/(u(3)^2+u(4)^2)
  Fcn2 : Fcn  Expr=u(1)*u(3)+u(2)*u(4)
  Gain : Gain  Gain=1/JGFM
  Gain1 : Gain  Gain=DGFM
  Gain11 : Gain  Gain=1/(2*pi)
  Gain12 : Gain  Gain=KPLlimit
  Gain13 : Gain  Gain=KILlimit
  Gain15 : Gain  Gain=W0
  Gain2 : Gain  Gain=W0
  Gain4 : Gain  Gain=1/LG
  Gain5 : Gain  Gain=-1/LG
  I1 : Constant  Value=0
  I3 : Constant  Value=0
  Integrator : Integrator
  Integrator1 : Integrator  InitialCondition=theta0
  Integrator6 : Integrator
  Integrator8 : Integrator  InitialCondition=theta0
  Mux{1..5,7,13,18..19} (9 alike) : Mux  Inputs=2
  Mux11 : Mux  Inputs=3
  Mux6 : Mux
  Park to Clarke Angle Transform2 : eeTransforms/Park to Clarke Angle Transform  AxisAlignment=D-axis
      settings: SourceProductBaseCode=PS
  Park to Clarke Angle Transform4 : eeTransforms/Park to Clarke Angle Transform  AxisAlignment=D-axis
      settings: SourceProductBaseCode=PS
  Pref : Constant  Value=Pref
  Product2 : Product
  Relay2 : Relay  OnSwitchValue=Plimit  OffSwitchValue=-1  OnOutputValue=1.1
  Scope{,1..3,5..8,13,15} (10 alike) : Scope
  Sum : Sum  Inputs=++--
  Sum of Elements : Sum  Inputs=+
  Sum15 : Sum  Inputs=|++
  Sum2 : Sum  Inputs=+-  SaturateOnIntegerOverflow=on
  Sum3 : Sum  Inputs=+-  SaturateOnIntegerOverflow=on
  Switch3 : Switch  Criteria=u2 > Threshold  Threshold=1.
  Terminator{1..3,5,8} (5 alike) : Terminator
  Ixy : Outport
  f : Outport  Port=2
  P : Outport  Port=3
  wires:
  Integrator1/1 -> [thetagfm], Scope1/1
  Gain/1 -> Integrator/1
  Integrator/1 -> Gain2/1, Scope/1, Gain1/1  "p.u."
  Fcn2/1 -> Sum/3, [P], Scope2/1
  Sum/1 -> Gain/1
  Vxy/1 -> [Vxy]
  Gain2/1 -> Gain11/1, Integrator1/1
  Gain11/1 -> f/1
  Pref/1 -> Sum/1
  Mux11/1 -> Fcn1/1, Fcn/1
  Constant/1 -> Mux11/1
  Constant2/1 -> Mux11/2
  Mux13/1 -> Scope13/1, [Idqref2]
  Integrator6/1 -> Sum15/2
  Gain13/1 -> Integrator6/1
  Demux4/1 -> Terminator5/1
  Gain15/1 -> Integrator8/1
  [Vdq] -> Demux4/1
  Demux4/2 -> Gain13/1, Gain12/1
  Integrator8/1 -> Scope15/1, [thetagfl]
  Gain12/1 -> Sum15/1
  Fcn/1 -> Mux13/1
  Fcn1/1 -> Mux13/2
  [Vdq] -> Mux11/3
  Sum15/1 -> [wpll], Gain15/1
  Gain1/1 -> Sum/4
  step/1 -> Sum/2
  Demux8/3 -> Terminator8/1
  Mux18/1 -> [Ixy2]
  Park to Clarke Angle Transform4/1 -> Demux8/1  "Ixy"
  Demux8/2 -> Mux18/2
  Demux8/1 -> Mux18/1
  [Idqref2] -> Mux19/1
  Constant8/1 -> Mux19/2
  Mux19/1 -> Park to Clarke Angle Transform4/1
  [thetagfl] -> Park to Clarke Angle Transform4/2
  [P] -> Abs1/1
  Abs1/1 -> Relay2/1
  Relay2/1 -> Scope6/1, Switch3/2
  [Ixy2] -> Switch3/1
  [Ixy] -> Switch3/3
  Switch3/1 -> [IOxy], Ixy/1
  [Vxy] -> Mux2/1
  Constant1/1 -> Mux2/2
  Mux2/1 -> Clarke to Park Angle Transform1/1
  [thetagfl] -> Clarke to Park Angle Transform1/2
  Demux1/3 -> Terminator1/1
  Mux1/1 -> Scope7/1, [Vdq]
  Clarke to Park Angle Transform1/1 -> Demux1/1  "Vxy"
  Demux1/2 -> Mux1/2
  Demux1/1 -> Mux1/1
  Constant3/1 -> Sum2/1
  [Vq] -> Scope5/1, Sum2/2
  Sum2/1 -> Gain4/1
  Gain4/1 -> [Id]
  Sum3/1 -> Gain5/1
  Constant4/1 -> Sum3/1
  [Vd] -> Sum3/2
  Gain5/1 -> [Iq]
  Demux2/3 -> Terminator2/1
  Demux3/1 -> [Vd]
  [thetagfm] -> Clarke to Park Angle Transform2/2
  Park to Clarke Angle Transform2/1 -> Demux2/1  "Vxy"
  Demux2/2 -> Mux5/2
  Mux4/1 -> Park to Clarke Angle Transform2/1
  Demux3/2 -> [Vq]
  Demux3/3 -> Terminator3/1
  I3/1 -> Mux7/2
  Demux2/1 -> Mux5/1
  Clarke to Park Angle Transform2/1 -> Demux3/1
  Mux5/1 -> [Ixy], Scope3/1
  [thetagfm] -> Park to Clarke Angle Transform2/2
  [Vxy] -> Mux7/1
  Mux7/1 -> Clarke to Park Angle Transform2/1
  [Id] -> Mux3/1
  [Iq] -> Mux3/2
  Mux3/1 -> Mux4/1
  I1/1 -> Mux4/2
  [Id] -> Mux6/3
  [Vd] -> Mux6/1
  Mux6/1 -> Fcn2/1
  [Vq] -> Mux6/2
  [Iq] -> Mux6/4
  [Vxy] -> Product2/1
  Product2/1 -> Sum of Elements/1
  [IOxy] -> Product2/2
  Sum of Elements/1 -> P/1, Scope8/1

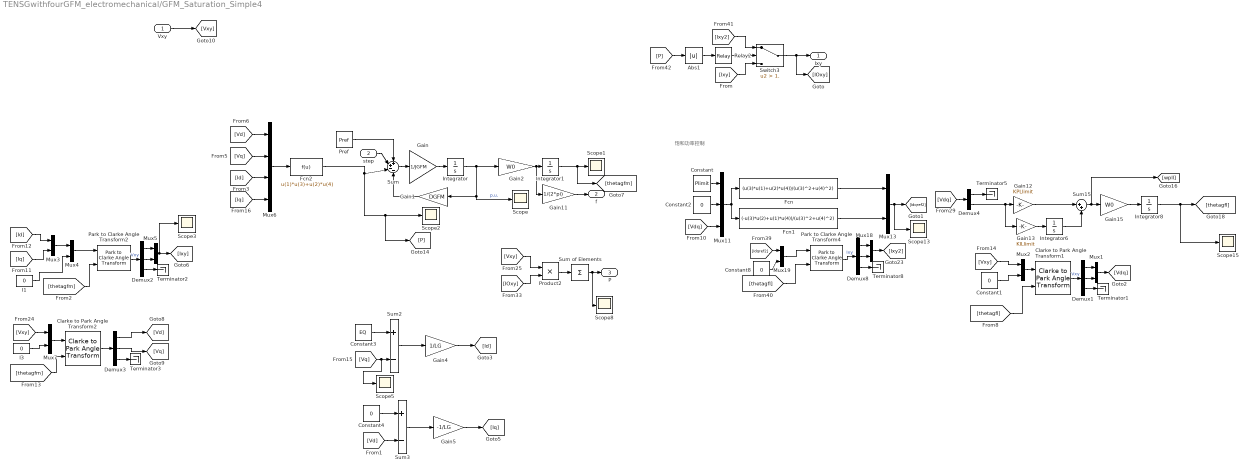
== system TENSGwithfourGFM_electromechanical/GFM_Saturation_Simple4 ==
  note: 饱和功率控制
  Vxy : Inport
  step : Inport  Port=2
  Abs1 : Abs
  Clarke to Park Angle Transform1 : eeTransforms/Clarke to Park Angle Transform  AxisAlignment=D-axis
      settings: SourceProductBaseCode=PS
  Clarke to Park Angle Transform2 : eeTransforms/Clarke to Park Angle Transform  AxisAlignment=D-axis
      settings: SourceProductBaseCode=PS
  Constant : Constant  Value=Plimit
  Constant{1..2,4,8} (4 alike) : Constant  Value=0
  Constant3 : Constant  Value=EQ
  Demux{1..3,8} (4 alike) : Demux  Outputs=3
  Demux4 : Demux  Outputs=2
  Fcn : Fcn  Expr=(u(3)*u(1)+u(2)*u(4))/(u(3)^2+u(4)^2)
  Fcn1 : Fcn  Expr=(-u(3)*u(2)+u(1)*u(4))/(u(3)^2+u(4)^2)
  Fcn2 : Fcn  Expr=u(1)*u(3)+u(2)*u(4)
  Gain : Gain  Gain=1/JGFM
  Gain1 : Gain  Gain=DGFM
  Gain11 : Gain  Gain=1/(2*pi)
  Gain12 : Gain  Gain=KPLlimit
  Gain13 : Gain  Gain=KILlimit
  Gain15 : Gain  Gain=W0
  Gain2 : Gain  Gain=W0
  Gain4 : Gain  Gain=1/LG
  Gain5 : Gain  Gain=-1/LG
  I1 : Constant  Value=0
  I3 : Constant  Value=0
  Integrator : Integrator
  Integrator1 : Integrator  InitialCondition=theta0
  Integrator6 : Integrator
  Integrator8 : Integrator  InitialCondition=theta0
  Mux{1..5,7,13,18..19} (9 alike) : Mux  Inputs=2
  Mux11 : Mux  Inputs=3
  Mux6 : Mux
  Park to Clarke Angle Transform2 : eeTransforms/Park to Clarke Angle Transform  AxisAlignment=D-axis
      settings: SourceProductBaseCode=PS
  Park to Clarke Angle Transform4 : eeTransforms/Park to Clarke Angle Transform  AxisAlignment=D-axis
      settings: SourceProductBaseCode=PS
  Pref : Constant  Value=Pref
  Product2 : Product
  Relay2 : Relay  OnSwitchValue=Plimit  OffSwitchValue=0  OnOutputValue=1.1
  Scope{,1..3,5,8,13,15} (8 alike) : Scope
  Sum : Sum  Inputs=++--
  Sum of Elements : Sum  Inputs=+
  Sum15 : Sum  Inputs=|++
  Sum2 : Sum  Inputs=+-  SaturateOnIntegerOverflow=on
  Sum3 : Sum  Inputs=+-  SaturateOnIntegerOverflow=on
  Switch3 : Switch  Criteria=u2 > Threshold  Threshold=1.
  Terminator{1..3,5,8} (5 alike) : Terminator
  Ixy : Outport
  f : Outport  Port=2
  P : Outport  Port=3
  wires:
  Integrator1/1 -> [thetagfm], Scope1/1
  Gain/1 -> Integrator/1
  Integrator/1 -> Gain2/1, Scope/1, Gain1/1  "p.u."
  Fcn2/1 -> Sum/3, [P], Scope2/1
  Sum/1 -> Gain/1
  Vxy/1 -> [Vxy]
  Gain2/1 -> Gain11/1, Integrator1/1
  Gain11/1 -> f/1
  Pref/1 -> Sum/1
  Mux11/1 -> Fcn1/1, Fcn/1
  Constant/1 -> Mux11/1
  Constant2/1 -> Mux11/2
  Mux13/1 -> Scope13/1, [Idqref2]
  Integrator6/1 -> Sum15/2
  Gain13/1 -> Integrator6/1
  Demux4/1 -> Terminator5/1
  Gain15/1 -> Integrator8/1
  [Vdq] -> Demux4/1
  Demux4/2 -> Gain13/1, Gain12/1
  Integrator8/1 -> Scope15/1, [thetagfl]
  Gain12/1 -> Sum15/1
  Fcn/1 -> Mux13/1
  Fcn1/1 -> Mux13/2
  [Vdq] -> Mux11/3
  Sum15/1 -> [wpll], Gain15/1
  Gain1/1 -> Sum/4
  step/1 -> Sum/2
  Demux8/3 -> Terminator8/1
  Mux18/1 -> [Ixy2]
  Park to Clarke Angle Transform4/1 -> Demux8/1  "Ixy"
  Demux8/2 -> Mux18/2
  Demux8/1 -> Mux18/1
  [Idqref2] -> Mux19/1
  Constant8/1 -> Mux19/2
  Mux19/1 -> Park to Clarke Angle Transform4/1
  [thetagfl] -> Park to Clarke Angle Transform4/2
  [P] -> Abs1/1
  Abs1/1 -> Relay2/1
  Relay2/1 -> Switch3/2
  [Ixy2] -> Switch3/1
  [Ixy] -> Switch3/3
  Switch3/1 -> [IOxy], Ixy/1
  [Vxy] -> Mux2/1
  Constant1/1 -> Mux2/2
  Mux2/1 -> Clarke to Park Angle Transform1/1
  [thetagfl] -> Clarke to Park Angle Transform1/2
  Demux1/3 -> Terminator1/1
  Mux1/1 -> [Vdq]
  Clarke to Park Angle Transform1/1 -> Demux1/1  "Vxy"
  Demux1/2 -> Mux1/2
  Demux1/1 -> Mux1/1
  Constant3/1 -> Sum2/1
  [Vq] -> Scope5/1, Sum2/2
  Sum2/1 -> Gain4/1
  Gain4/1 -> [Id]
  Sum3/1 -> Gain5/1
  Constant4/1 -> Sum3/1
  [Vd] -> Sum3/2
  Gain5/1 -> [Iq]
  Demux2/3 -> Terminator2/1
  Demux3/1 -> [Vd]
  [thetagfm] -> Clarke to Park Angle Transform2/2
  Park to Clarke Angle Transform2/1 -> Demux2/1  "Vxy"
  Demux2/2 -> Mux5/2
  Mux4/1 -> Park to Clarke Angle Transform2/1
  Demux3/2 -> [Vq]
  Demux3/3 -> Terminator3/1
  I3/1 -> Mux7/2
  Demux2/1 -> Mux5/1
  Clarke to Park Angle Transform2/1 -> Demux3/1
  Mux5/1 -> [Ixy], Scope3/1
  [thetagfm] -> Park to Clarke Angle Transform2/2
  [Vxy] -> Mux7/1
  Mux7/1 -> Clarke to Park Angle Transform2/1
  [Id] -> Mux3/1
  [Iq] -> Mux3/2
  Mux3/1 -> Mux4/1
  I1/1 -> Mux4/2
  [Id] -> Mux6/3
  [Vd] -> Mux6/1
  Mux6/1 -> Fcn2/1
  [Vq] -> Mux6/2
  [Iq] -> Mux6/4
  [IOxy] -> Product2/2
  Product2/1 -> Sum of Elements/1
  Sum of Elements/1 -> Scope8/1, P/1
  [Vxy] -> Product2/1

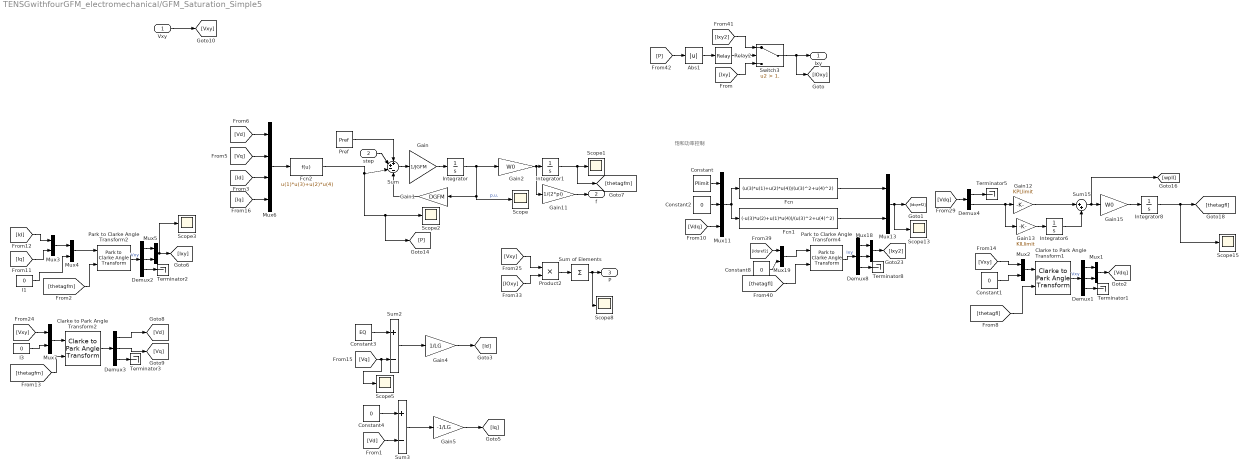
== system TENSGwithfourGFM_electromechanical/GFM_Saturation_Simple5 ==
  note: 饱和功率控制
  Vxy : Inport
  step : Inport  Port=2
  Abs1 : Abs
  Clarke to Park Angle Transform1 : eeTransforms/Clarke to Park Angle Transform  AxisAlignment=D-axis
      settings: SourceProductBaseCode=PS
  Clarke to Park Angle Transform2 : eeTransforms/Clarke to Park Angle Transform  AxisAlignment=D-axis
      settings: SourceProductBaseCode=PS
  Constant : Constant  Value=Plimit
  Constant{1..2,4,8} (4 alike) : Constant  Value=0
  Constant3 : Constant  Value=EQ
  Demux{1..3,8} (4 alike) : Demux  Outputs=3
  Demux4 : Demux  Outputs=2
  Fcn : Fcn  Expr=(u(3)*u(1)+u(2)*u(4))/(u(3)^2+u(4)^2)
  Fcn1 : Fcn  Expr=(-u(3)*u(2)+u(1)*u(4))/(u(3)^2+u(4)^2)
  Fcn2 : Fcn  Expr=u(1)*u(3)+u(2)*u(4)
  Gain : Gain  Gain=1/JGFM
  Gain1 : Gain  Gain=DGFM
  Gain11 : Gain  Gain=1/(2*pi)
  Gain12 : Gain  Gain=KPLlimit
  Gain13 : Gain  Gain=KILlimit
  Gain15 : Gain  Gain=W0
  Gain2 : Gain  Gain=W0
  Gain4 : Gain  Gain=1/LG
  Gain5 : Gain  Gain=-1/LG
  I1 : Constant  Value=0
  I3 : Constant  Value=0
  Integrator : Integrator
  Integrator1 : Integrator  InitialCondition=theta0
  Integrator6 : Integrator
  Integrator8 : Integrator  InitialCondition=theta0
  Mux{1..5,7,13,18..19} (9 alike) : Mux  Inputs=2
  Mux11 : Mux  Inputs=3
  Mux6 : Mux
  Park to Clarke Angle Transform2 : eeTransforms/Park to Clarke Angle Transform  AxisAlignment=D-axis
      settings: SourceProductBaseCode=PS
  Park to Clarke Angle Transform4 : eeTransforms/Park to Clarke Angle Transform  AxisAlignment=D-axis
      settings: SourceProductBaseCode=PS
  Pref : Constant  Value=Pref
  Product2 : Product
  Relay2 : Relay  OnSwitchValue=Plimit  OffSwitchValue=0  OnOutputValue=1.1
  Scope{,1..3,5,8,13,15} (8 alike) : Scope
  Sum : Sum  Inputs=++--
  Sum of Elements : Sum  Inputs=+
  Sum15 : Sum  Inputs=|++
  Sum2 : Sum  Inputs=+-  SaturateOnIntegerOverflow=on
  Sum3 : Sum  Inputs=+-  SaturateOnIntegerOverflow=on
  Switch3 : Switch  Criteria=u2 > Threshold  Threshold=1.
  Terminator{1..3,5,8} (5 alike) : Terminator
  Ixy : Outport
  f : Outport  Port=2
  P : Outport  Port=3
  wires:
  Integrator1/1 -> [thetagfm], Scope1/1
  Gain/1 -> Integrator/1
  Integrator/1 -> Gain2/1, Scope/1, Gain1/1  "p.u."
  Fcn2/1 -> Sum/3, [P], Scope2/1
  Sum/1 -> Gain/1
  Vxy/1 -> [Vxy]
  Gain2/1 -> Gain11/1, Integrator1/1
  Gain11/1 -> f/1
  Pref/1 -> Sum/1
  Mux11/1 -> Fcn1/1, Fcn/1
  Constant/1 -> Mux11/1
  Constant2/1 -> Mux11/2
  Mux13/1 -> Scope13/1, [Idqref2]
  Integrator6/1 -> Sum15/2
  Gain13/1 -> Integrator6/1
  Demux4/1 -> Terminator5/1
  Gain15/1 -> Integrator8/1
  [Vdq] -> Demux4/1
  Demux4/2 -> Gain13/1, Gain12/1
  Integrator8/1 -> Scope15/1, [thetagfl]
  Gain12/1 -> Sum15/1
  Fcn/1 -> Mux13/1
  Fcn1/1 -> Mux13/2
  [Vdq] -> Mux11/3
  Sum15/1 -> [wpll], Gain15/1
  Gain1/1 -> Sum/4
  step/1 -> Sum/2
  Demux8/3 -> Terminator8/1
  Mux18/1 -> [Ixy2]
  Park to Clarke Angle Transform4/1 -> Demux8/1  "Ixy"
  Demux8/2 -> Mux18/2
  Demux8/1 -> Mux18/1
  [Idqref2] -> Mux19/1
  Constant8/1 -> Mux19/2
  Mux19/1 -> Park to Clarke Angle Transform4/1
  [thetagfl] -> Park to Clarke Angle Transform4/2
  [P] -> Abs1/1
  Abs1/1 -> Relay2/1
  Relay2/1 -> Switch3/2
  [Ixy2] -> Switch3/1
  [Ixy] -> Switch3/3
  Switch3/1 -> [IOxy], Ixy/1
  [Vxy] -> Mux2/1
  Constant1/1 -> Mux2/2
  Mux2/1 -> Clarke to Park Angle Transform1/1
  [thetagfl] -> Clarke to Park Angle Transform1/2
  Demux1/3 -> Terminator1/1
  Mux1/1 -> [Vdq]
  Clarke to Park Angle Transform1/1 -> Demux1/1  "Vxy"
  Demux1/2 -> Mux1/2
  Demux1/1 -> Mux1/1
  Constant3/1 -> Sum2/1
  [Vq] -> Scope5/1, Sum2/2
  Sum2/1 -> Gain4/1
  Gain4/1 -> [Id]
  Sum3/1 -> Gain5/1
  Constant4/1 -> Sum3/1
  [Vd] -> Sum3/2
  Gain5/1 -> [Iq]
  Demux2/3 -> Terminator2/1
  Demux3/1 -> [Vd]
  [thetagfm] -> Clarke to Park Angle Transform2/2
  Park to Clarke Angle Transform2/1 -> Demux2/1  "Vxy"
  Demux2/2 -> Mux5/2
  Mux4/1 -> Park to Clarke Angle Transform2/1
  Demux3/2 -> [Vq]
  Demux3/3 -> Terminator3/1
  I3/1 -> Mux7/2
  Demux2/1 -> Mux5/1
  Clarke to Park Angle Transform2/1 -> Demux3/1
  Mux5/1 -> [Ixy], Scope3/1
  [thetagfm] -> Park to Clarke Angle Transform2/2
  [Vxy] -> Mux7/1
  Mux7/1 -> Clarke to Park Angle Transform2/1
  [Id] -> Mux3/1
  [Iq] -> Mux3/2
  Mux3/1 -> Mux4/1
  I1/1 -> Mux4/2
  [Id] -> Mux6/3
  [Vd] -> Mux6/1
  Mux6/1 -> Fcn2/1
  [Vq] -> Mux6/2
  [Iq] -> Mux6/4
  [IOxy] -> Product2/2
  Product2/1 -> Sum of Elements/1
  Sum of Elements/1 -> Scope8/1, P/1
  [Vxy] -> Product2/1

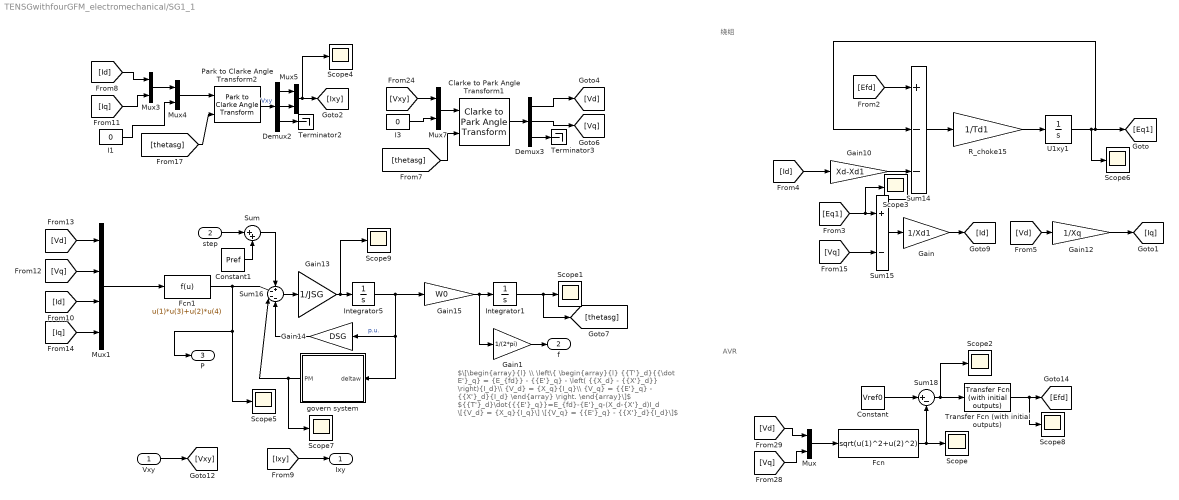
== system TENSGwithfourGFM_electromechanical/SG1_1 ==
  note: $\[\begin{array}{l} \\ \left\{ \begin{array}{l} {{T'}_d}{{\dot E'}_q} = {E_{fd}} - {{E'}_q} - \left( {{X_d} - {{X'}_d}} \right){I_d}\\ {V_d} = {X_q}{I_q}\\ {V_q} = {{E'}_q} - {{X'}_d}{I_d} \end{array} \right. \end{array}\]$ ${{T'}_d}\dot{{{E'}_q}}=E_{fd}-{E'}_q-(X_d-{X'}_d)I_d \[{V_d} = {X_q}{I_q}\] \[{V_q} = {{E'}_q} - {{X'}_d}{I_d}\]$
  note: AVR
  note: 绕组
  Vxy : Inport
  step : Inport  Port=2
  Clarke to Park Angle Transform1 : eeTransforms/Clarke to Park Angle Transform  AxisAlignment=D-axis
      settings: SourceProductBaseCode=PS
  Constant : Constant  Value=Vref0
  Constant1 : Constant  Value=Pref
  Demux2 : Demux  Outputs=3
  Demux3 : Demux  Outputs=3
  Fcn : Fcn  Expr=sqrt(u(1)^2+u(2)^2)
  Fcn1 : Fcn  Expr=u(1)*u(3)+u(2)*u(4)
  Gain : Gain  Gain=1/Xd1
  Gain1 : Gain  Gain=1/(2*pi)
  Gain10 : Gain  Gain=Xd-Xd1
  Gain12 : Gain  Gain=1/Xq
  Gain13 : Gain  Gain=1/JSG
  Gain14 : Gain  Gain=DSG
  Gain15 : Gain  Gain=W0
  I1 : Constant  Value=0
  I3 : Constant  Value=0
  Integrator1 : Integrator  InitialCondition=theta0
  Integrator5 : Integrator
  Mux{,3..5,7} (5 alike) : Mux  Inputs=2
  Mux1 : Mux
  Park to Clarke Angle Transform2 : eeTransforms/Park to Clarke Angle Transform  AxisAlignment=D-axis
      settings: SourceProductBaseCode=PS
  R_choke15 : Gain  Gain=1/Td1  SaturateOnIntegerOverflow=on  OutDataTypeStr=Inherit: Same as input  ParamDataTypeStr=Inherit: Same as input
  Scope{,1..9} (10 alike) : Scope
  Sum : Sum  Inputs=|++
  Sum14 : Sum  Inputs=+--  SaturateOnIntegerOverflow=on
  Sum15 : Sum  Inputs=+-  SaturateOnIntegerOverflow=on
  Sum16 : Sum  Inputs=+---
  Sum18 : Sum  Inputs=|+-
  Terminator2 : Terminator
  Terminator3 : Terminator
  Transfer Fcn (with initial outputs) : simulink_extras/Additional Linear/Transfer Fcn (with initial outputs)  N=[KAVR]  D=[TAVR 1]  Y0=Efd0  U0=0
  U1xy1 : Integrator  InitialCondition=Eq10
  govern system : Subsystem
  Ixy : Outport
  f : Outport  Port=2
  P : Outport  Port=3
  wires:
  Integrator1/1 -> [thetasg], Scope1/1
  Gain15/1 -> Gain1/1, Integrator1/1
  [Efd] -> Sum14/1
  Sum14/1 -> R_choke15/1
  R_choke15/1 -> U1xy1/1
  U1xy1/1 -> Scope6/1, [Eq1], Sum14/2
  [Id] -> Gain10/1
  Gain10/1 -> Sum14/3
  [Eq1] -> Scope3/1, Sum15/1
  [Vq] -> Sum15/2
  Sum15/1 -> Gain/1
  [Vd] -> Gain12/1
  Gain12/1 -> [Iq]
  govern system/1(PM) -> Scope7/1, Sum16/3
  Gain13/1 -> Scope9/1, Integrator5/1
  Gain14/1 -> Sum16/4
  Sum16/1 -> Gain13/1
  Integrator5/1 -> Gain15/1, govern system/1(deltaw), Gain14/1  "p.u."
  Fcn1/1 -> P/1, Scope5/1, Sum16/2
  Sum18/1 -> Transfer Fcn (with initial outputs)/1, Scope2/1
  [Vd] -> Mux/1
  [Vq] -> Mux/2
  Mux/1 -> Fcn/1
  Constant/1 -> Sum18/1
  Transfer Fcn (with initial outputs)/1 -> Scope8/1, [Efd]
  [Vq] -> Mux1/2
  [Vd] -> Mux1/1
  [Id] -> Mux1/3
  [Iq] -> Mux1/4
  Mux1/1 -> Fcn1/1
  [Iq] -> Mux3/2
  [Id] -> Mux3/1
  Mux4/1 -> Park to Clarke Angle Transform2/1
  I1/1 -> Mux4/2
  Mux3/1 -> Mux4/1
  Demux2/3 -> Terminator2/1
  Demux2/2 -> Mux5/2
  Mux5/1 -> [Ixy], Scope4/1
  [thetasg] -> Park to Clarke Angle Transform2/2
  Park to Clarke Angle Transform2/1 -> Demux2/1  "Vxy"
  Demux2/1 -> Mux5/1
  Vxy/1 -> [Vxy]
  [Ixy] -> Ixy/1
  Fcn/1 -> Scope/1, Sum18/2
  Mux7/1 -> Clarke to Park Angle Transform1/1
  Clarke to Park Angle Transform1/1 -> Demux3/1
  [Vxy] -> Mux7/1
  [thetasg] -> Clarke to Park Angle Transform1/2
  I3/1 -> Mux7/2
  Demux3/3 -> Terminator3/1
  Demux3/2 -> [Vq]
  Demux3/1 -> [Vd]
  Gain/1 -> [Id]
  Gain1/1 -> f/1
  Sum/1 -> Sum16/1
  step/1 -> Sum/1
  Constant1/1 -> Sum/2
